simulink model "model_mcp_boost_pressure"  (R2020a)
settings: Solver=ode4  StartTime=0.0  StopTime=30  FixedStep=0.2  RelTol=1e-3
InitFcn:
  | load pot.mat;
  | load rpm.mat;
model workspace (MAT data in the model file):
  k_boost_pressure = 0
  k_boost_pressure_error = -5
settings Model: Creator=victo  LastModifiedBy=suina
settings DataIOCC: SaveOutput=off  SaveTime=off
settings OptimizationCC: DefaultParameterBehavior=Inlined  EnhancedBackFolding=on  PassReuseOutputArgsAs=Individual arguments  ZeroExternalMemoryAtStartup=off  ZeroInternalMemoryAtStartup=off  OptimizeBlockOrder=speed  DifferentSizesBufferReuse=on  OptimizationCustomize=off  EfficientTunableParamExpr=on
settings DebuggingCC: UnderspecifiedInitializationDetection=Classic  MergeDetectMultiDrivingBlocksExec=none  ParameterTunabilityLossMsg=error
settings ModelReferenceCC: PropagateSignalLabelsOutOfModel=off
settings SFSimCC: MATLABDynamicMemAlloc=off
settings RTWCC: SystemTargetFile=ert.tlc  TemplateMakefile=ert_default_tmf  TargetLang=C++
settings CodeAppCC: ForceParamTrailComments=on  IgnoreCustomStorageClasses=off  OperatorAnnotations=on  SimulinkDataObjDesc=on  SFDataObjDesc=on  InsertBlockDesc=on
settings ERTTargetCC: TargetLangStandard=C++03 (ISO)  GenerateSampleERTMain=on  MultiInstanceERTCode=on  CodeInterfacePackaging=C++ class  InlinedParameterPlacement=NonHierarchical  RootIOFormat=Structure reference  ERTCustomFileTemplate=example_file_process.tlc

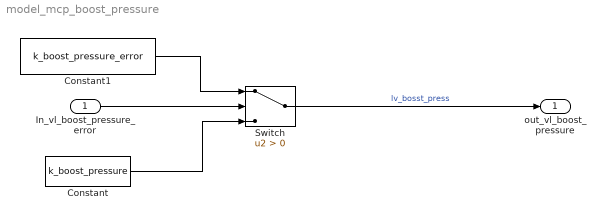
== system model_mcp_boost_pressure ==
  In_vl_boost_pressure_error : Inport  RequirementInfo={} %GIDa_6570dab6_0d32_4b4b_821a_ae2d57fd705b  OutDataTypeStr=boolean  PortDimensions=1
  Constant : Constant  RequirementInfo={} %GIDa_847df1cb_0b24_4391_b2a8_aef8c634d2ce  Value=k_boost_pressure  OutDataTypeStr=int16
  Constant1 : Constant  RequirementInfo={} %GIDa_0c01cf73_8e93_4c7f_a367_86bd7bef3901  Value=k_boost_pressure_error  OutDataTypeStr=int16
  Switch : Switch  RequirementInfo={} %GIDa_8389b724_d565_4699_a257_bca7e76e527a  Criteria=u2 > Threshold
  out_vl_boost_pressure : Outport  RequirementInfo={} %GIDa_4b6c8a65_8a9c_443d_a57d_f4adab4fa5d9  OutDataTypeStr=int16  PortDimensions=1  SampleTime=[0.20000000000000001,0]
  wires:
  In_vl_boost_pressure_error/1 -> Switch/2
  Switch/1 -> out_vl_boost_pressure/1  "lv_bosst_press"
  Constant1/1 -> Switch/1
  Constant/1 -> Switch/3
